simulink model "Winch_All_Controllers_with_Noise"  (R2016a)
settings: Solver=VariableStepAuto  SolverMode=SingleTasking  StartTime=0.0  StopTime=500  RelTol=1e-3
undefined symbols (not defined in the file or in its folder): K
libraries: mpclib x1, simulink x1
settings Model: Creator=shrenikzinage  LastModifiedBy=shrenikzinage
settings DataIOCC: SaveFormat=Array
settings DebuggingCC: SFUnexpectedBacktrackingDiag=error  SFNoUnconditionalDefaultTransitionDiag=error
settings SFSimCC: SimUseLocalCustomCode=on
settings RTWCC: RTWUseLocalCustomCode=on
settings GRTTargetCC: TargetLangStandard=C99 (ISO)  GeneratePreprocessorConditionals=Use local settings
settings ConfigComp: CovMetricSettings=dwe  CovHtmlReporting=off  CovSaveCumulativeToWorkspaceVar=off  CovSaveSingleToWorkspaceVar=off  CovExternalEMLEnable=on

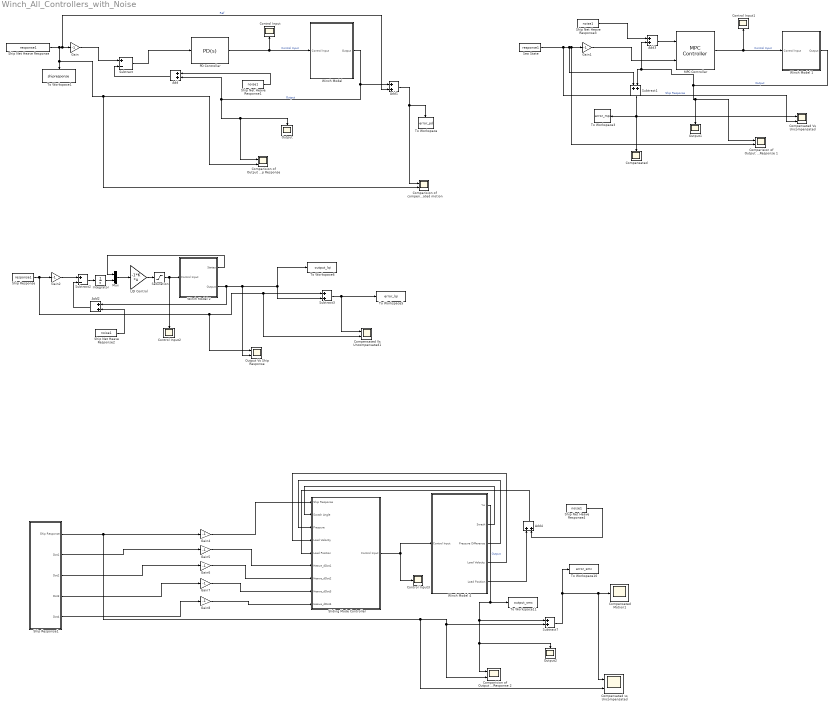
== system Winch_All_Controllers_with_Noise ==
  Add{,1..4} (5 alike) : Sum
  "Comparision of Output and Ship Response " : Scope  NumInputPorts=2
  Comparision of Output and Ship Response 1 : Scope  NumInputPorts=2
  Comparision of Output and Ship Response 2 : Scope  NumInputPorts=2
  Comparision of compensated and uncompensated motion : Scope  NumInputPorts=2
  Compensated : Scope
  Compensated Motion1 : Scope
  Compensated Vs Uncompensated : Scope  NumInputPorts=2
  Compensated Vs Uncompensated1 : Scope  NumInputPorts=2
  "Compensated vs Uncompensated " : Scope  NumInputPorts=2
  Control Input{,1..3} (4 alike) : Scope
  Gain{,1..2,4..8} (8 alike) : Gain  Gain=-1
  Integrator : Integrator
  LQI Control : Gain  Gain=-1*K  Multiplication=Matrix(K*u) (u vector)
  MPC Controller : mpclib/MPC Controller  SCDEnableBlockLinearizationSpecification=on  mpcobj=mpc1  is_multiple=0  enable_value=0  return_u0=off  updateMPCinCallerWorkspace=on  md_inport=off  mv_inport=off  uref_inport=off  cost_outport=off  return_sequence=off  return_qpstatus=off  return_xseq=off  return_state=off  return_ovseq=off  state_inport=off  umin_inport=off  umax_inport=off  ymin_inport=off  ymax_inport=off  cc_inport=off  ywt_inport=off  uwt_inport=off  duwt_inport=off  rhoeps_inport=off  pm_inport=off  MaximumP=10  HorizonChoice=FixedHorizon  n_ts=0.05  n_p=20  n_mv=1  n_md=0  n_ud=0  n_mo=1  n_uo=0  BlockDataType=double  SampleTimeInherited=off  switch_inport=off
  Mux : Mux  Inputs=2
  Output : Scope
  Output Vs Ship Response : Scope  NumInputPorts=2
  Output1 : Scope
  Output2 : Scope
  "PD Controller " : simulink/Continuous/PID Controller  Controller=PD  Form=Parallel  TimeDomain=Continuous-time  SampleTime=-1  IntegratorMethod=Forward Euler  FilterMethod=Forward Euler  ControllerParametersSource=internal  P=5.86  I=0.711  D=5.46  UseFilter=on  N=33.33  InitialConditionSource=internal  InitialConditionForIntegrator=0  InitialConditionForFilter=0  DifferentiatorICPrevScaledInput=0  ExternalReset=none  TrackingMode=off  Kt=1  LimitOutput=on  UpperSaturationLimit=200  LowerSaturationLimit=-200  LinearizeAsGain=on  AntiWindupMode=none  Kb=1  POutMin=[]  POutMax=[]  IOutMin=[]  IOutMax=[]  DOutMin=[]  DOutMax=[]  NOutMin=[]  NOutMax=[]  SumOutMin=[]  SumOutMax=[]  SaturationOutMin=[]  SaturationOutMax=[]  PParamMin=[]  PParamMax=[]  IParamMin=[]  IParamMax=[]  DParamMin=[]  DParamMax=[]  NParamMin=[]  NParamMax=[]  KbParamMin=[]  KbParamMax=[]  KtParamMin=[]  KtParamMax=[]  KbOutMin=[]  KbOutMax=[]  KtOutMin=[]  KtOutMax=[]  IntegratorOutMin=[]  IntegratorOutMax=[]  FilterOutMin=[]  FilterOutMax=[]  SumI1OutMin=[]  SumI1OutMax=[]  SumI2OutMin=[]  SumI2OutMax=[]  SumI3OutMin=[]  SumI3OutMax=[]  SumDOutMin=[]  SumDOutMax=[]  DifferentiatorOutMin=[]  DifferentiatorOutMax=[]  IntegratorContinuousStateAttributes=''  IntegratorStateMustResolveToSignalObject=off  IntegratorRTWStateStorageClass=Auto  FilterContinuousStateAttributes=''  FilterStateMustResolveToSignalObject=off  FilterRTWStateStorageClass=Auto
  Saturation : Saturate  UpperLimit=200  LowerLimit=-200
  Sea State : FromWorkspace  VariableName=response1  SampleTime=0
  Ship Net Heave Response : FromWorkspace  VariableName=response1  SampleTime=0
  Ship Net Heave Response{1..4} (4 alike) : FromWorkspace  VariableName=noise1  SampleTime=0
  Ship Response : FromWorkspace  VariableName=response1  SampleTime=0
  Ship Response1 : Subsystem
  Sliding Mode Controller : Subsystem
  Subtract : Sum  Inputs=+-
  Subtract1 : Sum
  Subtract2 : Sum  Inputs=+-
  Subtract3 : Sum
  Subtract7 : Sum
  To Workspace : ToWorkspace  VariableName=error_pd  SampleTime=-1
  To Workspace1 : ToWorkspace  VariableName=shipresponse  SampleTime=-1
  To Workspace10 : ToWorkspace  VariableName=error_smc  SampleTime=-1
  To Workspace11 : ToWorkspace  VariableName=output_smc  SampleTime=-1
  To Workspace3 : ToWorkspace  VariableName=error_mpc  SampleTime=-1
      settings: Save2DSignal=2-D array (concatenate along first dimension)
  To Workspace5 : ToWorkspace  VariableName=error_lqi  SampleTime=-1
  To Workspace6 : ToWorkspace  VariableName=output_lqi  SampleTime=-1
  "Winch Model " : Subsystem
  Winch Model 1 : Subsystem
  Winch Model 2 : Subsystem
  Winch Model 4 : Subsystem
  wires:
  LQI Control/1 -> Saturation/1
  Saturation/1 -> Winch Model 2/1(Control Input), Control Input2/1
  Ship Response1/4(Dot3) -> Gain7/1
  Winch Model 4/2(Swash) -> Sliding Mode Controller/2(Swash Angle)
  Winch Model 4/1(Yw) -> Comparision of Output and Ship Response 2/1, Output2/1, Subtract7/1, To Workspace11/1  "Output"
  Subtract7/1 -> To Workspace10/1, "Compensated vs Uncompensated "/1, Compensated Motion1/1
  Mux/1 -> LQI Control/1
  Gain8/1 -> Sliding Mode Controller/9(Heave_dDot4)
  Gain1/1 -> MPC Controller/2
  Ship Response1/3(Dot2) -> Gain6/1
  Winch Model 2/1(States) -> Mux/1
  Ship Response1/2(Dot1) -> Gain5/1
  Winch Model 4/3(Pressure Difference) -> Sliding Mode Controller/3(Pressure)
  Ship Response1/1(Ship Response) -> Gain4/1, "Compensated vs Uncompensated "/2, Comparision of Output and Ship Response 2/2, Subtract7/2
  Gain7/1 -> Sliding Mode Controller/8(Heave_dDot3)
  Ship Response1/5(Dot4) -> Gain8/1
  Subtract/1 -> "PD Controller "/1
  Gain5/1 -> Sliding Mode Controller/6("Heave_dDot1 ")
  Ship Response/1 -> Output Vs Ship Response/1, Compensated Vs Uncompensated1/2, Subtract3/1, Gain2/1
  Gain2/1 -> Subtract2/1
  Subtract2/1 -> Integrator/1
  Winch Model 1/1("Output ") -> Add3/2, Subtract1/2, Comparision of Output and Ship Response 1/1, Output1/1  "Output"
  Winch Model 4/4(Load Velocity) -> Sliding Mode Controller/4(Load Velocity)
  "PD Controller "/1 -> "Winch Model "/1(Control Input), Control Input/1  "Control Input"
  Integrator/1 -> Mux/2
  Winch Model 2/2("Output ") -> Add2/1, Output Vs Ship Response/2, Subtract3/2, To Workspace6/1
  Subtract3/1 -> Compensated Vs Uncompensated1/1, To Workspace5/1
  Gain/1 -> Subtract/1
  Sea State/1 -> Compensated Vs Uncompensated/2, Subtract1/1, Comparision of Output and Ship Response 1/2, Gain1/1  "Ship Response"
  Ship Net Heave Response/1 -> "Comparision of Output and Ship Response "/2, Comparision of compensated and uncompensated motion/2, To Workspace1/1, Add1/2, Gain/1  "Ref"
  MPC Controller/1 -> Winch Model 1/1("Control Input "), Control Input1/1  "Control Input"
  Sliding Mode Controller/1(Control Input) -> Winch Model 4/1(Control Input), Control Input3/1
  "Winch Model "/1("Output ") -> Add/2, "Comparision of Output and Ship Response "/1, Output/1, Add1/1  "Output"
  Subtract1/1 -> To Workspace3/1, Compensated/1, Compensated Vs Uncompensated/1
  Gain4/1 -> Sliding Mode Controller/1(Ship Response)
  Gain6/1 -> Sliding Mode Controller/7(Heave_dDot2)
  Ship Net Heave Response1/1 -> Add/1
  Add/1 -> Subtract/2
  Add1/1 -> To Workspace/1, Comparision of compensated and uncompensated motion/1
  Ship Net Heave Response2/1 -> Add2/2
  Add2/1 -> Subtract2/2
  Ship Net Heave Response3/1 -> Add3/1
  Add3/1 -> MPC Controller/1
  Winch Model 4/5(Load Position) -> Add4/1
  Ship Net Heave Response4/1 -> Add4/2
  Add4/1 -> Sliding Mode Controller/5(Load Position)

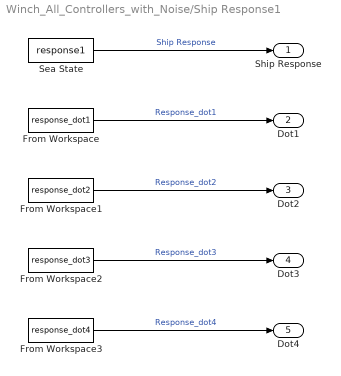
== system Winch_All_Controllers_with_Noise/Ship Response1 ==
  From Workspace : FromWorkspace  VariableName=response_dot1  SampleTime=0
  From Workspace1 : FromWorkspace  VariableName=response_dot2  SampleTime=0
  From Workspace2 : FromWorkspace  VariableName=response_dot3  SampleTime=0
  From Workspace3 : FromWorkspace  VariableName=response_dot4  SampleTime=0
  "Sea State " : FromWorkspace  VariableName=response1  SampleTime=0
  Ship Response : Outport
  Dot1 : Outport  Port=2
  Dot2 : Outport  Port=3
  Dot3 : Outport  Port=4
  Dot4 : Outport  Port=5
  wires:
  "Sea State "/1 -> Ship Response/1  "Ship Response"
  From Workspace3/1 -> Dot4/1  "Response_dot4"
  From Workspace1/1 -> Dot2/1  "Response_dot2"
  From Workspace2/1 -> Dot3/1  "Response_dot3"
  From Workspace/1 -> Dot1/1  "Response_dot1"

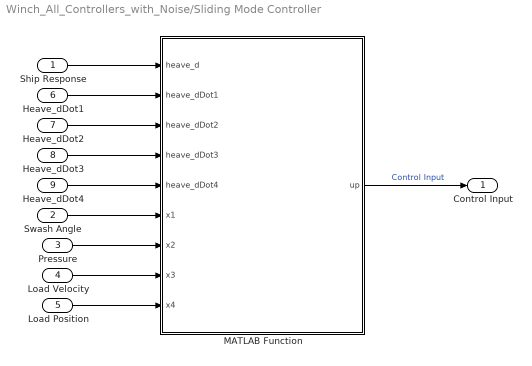
== system Winch_All_Controllers_with_Noise/Sliding Mode Controller ==
  Ship Response : Inport
  Swash Angle : Inport  Port=2
  Pressure : Inport  Port=3
  Load Velocity : Inport  Port=4
  Load Position : Inport  Port=5
  "Heave_dDot1 " : Inport  Port=6
  Heave_dDot2 : Inport  Port=7
  Heave_dDot3 : Inport  Port=8
  Heave_dDot4 : Inport  Port=9
  MATLAB Function : MATLAB Function  TreatAsAtomicUnit=on
  Control Input : Outport
  wires:
  Heave_dDot4/1 -> MATLAB Function/5(heave_dDot4)
  Ship Response/1 -> MATLAB Function/1(heave_d)
  MATLAB Function/1(up) -> Control Input/1  "Control Input"
  Heave_dDot2/1 -> MATLAB Function/3(heave_dDot2)
  Load Velocity/1 -> MATLAB Function/8(x3)
  Heave_dDot3/1 -> MATLAB Function/4(heave_dDot3)
  Load Position/1 -> MATLAB Function/9(x4)
  "Heave_dDot1 "/1 -> MATLAB Function/2(heave_dDot1)
  Swash Angle/1 -> MATLAB Function/6(x1)
  Pressure/1 -> MATLAB Function/7(x2)

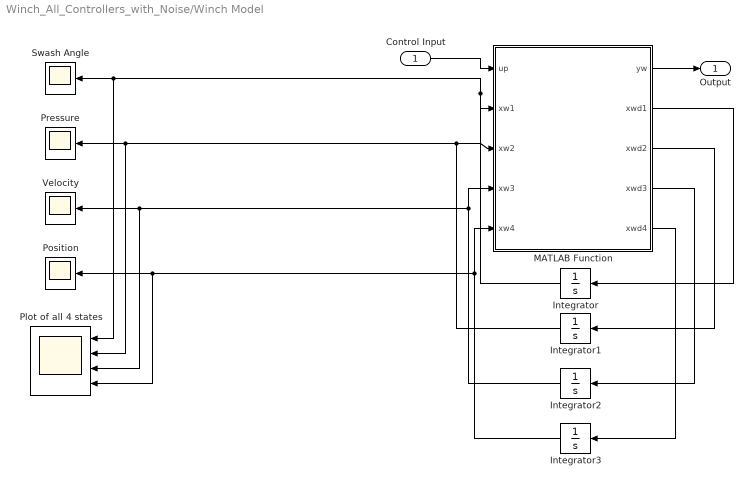
== system Winch_All_Controllers_with_Noise/Winch Model  ==
  Control Input : Inport
  Integrator : Integrator  InitialCondition=0.4  LimitOutput=on  UpperSaturationLimit=1  LowerSaturationLimit=-1  ContinuousStateAttributes='Swash'
  Integrator1 : Integrator  InitialCondition=188e5  UpperSaturationLimit=4e7  LowerSaturationLimit=-4e7  ContinuousStateAttributes='Pressure'
  Integrator2 : Integrator  ContinuousStateAttributes='Velocity'
  Integrator3 : Integrator  ContinuousStateAttributes='Position'
  MATLAB Function : MATLAB Function  TreatAsAtomicUnit=on
  Plot of all 4 states : Scope  NumInputPorts=4
  Position : Scope
  Pressure : Scope
  Swash Angle : Scope
  Velocity : Scope
  "Output " : Outport
  wires:
  Integrator2/1 -> MATLAB Function/4(xw3), Plot of all 4 states/3, Velocity/1
  MATLAB Function/4(xwd3) -> Integrator2/1
  MATLAB Function/3(xwd2) -> Integrator1/1
  Integrator/1 -> Plot of all 4 states/1, Swash Angle/1, MATLAB Function/2(xw1)
  MATLAB Function/2(xwd1) -> Integrator/1
  Integrator1/1 -> MATLAB Function/3(xw2), Plot of all 4 states/2, Pressure/1
  Integrator3/1 -> MATLAB Function/5(xw4), Plot of all 4 states/4, Position/1
  Control Input/1 -> MATLAB Function/1(up)
  MATLAB Function/5(xwd4) -> Integrator3/1
  MATLAB Function/1(yw) -> "Output "/1

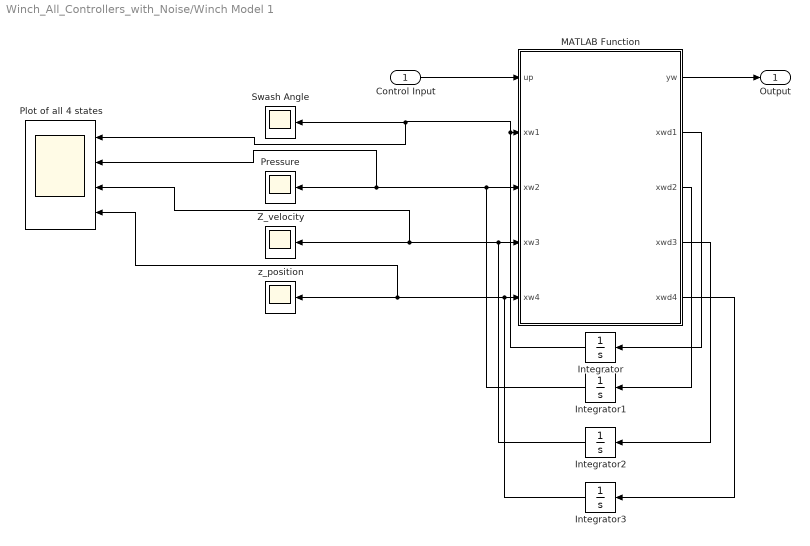
== system Winch_All_Controllers_with_Noise/Winch Model 1 ==
  "Control Input " : Inport
  Integrator : Integrator  InitialCondition=0.3  LimitOutput=on  UpperSaturationLimit=1  LowerSaturationLimit=-1
  Integrator1 : Integrator  InitialCondition=188e5  UpperSaturationLimit=5e7  LowerSaturationLimit=-5e7
  Integrator2 : Integrator
  Integrator3 : Integrator
  MATLAB Function : MATLAB Function  TreatAsAtomicUnit=on
  Plot of all 4 states : Scope  NumInputPorts=4
  Pressure : Scope
  Swash Angle : Scope
  Z_velocity : Scope
  z_position : Scope
  "Output " : Outport
  wires:
  MATLAB Function/1(yw) -> "Output "/1
  Integrator2/1 -> MATLAB Function/4(xw3), Z_velocity/1, Plot of all 4 states/3
  MATLAB Function/4(xwd3) -> Integrator2/1
  MATLAB Function/3(xwd2) -> Integrator1/1
  Integrator/1 -> Plot of all 4 states/1, Swash Angle/1, MATLAB Function/2(xw1)
  MATLAB Function/2(xwd1) -> Integrator/1
  Integrator1/1 -> MATLAB Function/3(xw2), Plot of all 4 states/2, Pressure/1
  Integrator3/1 -> MATLAB Function/5(xw4), Plot of all 4 states/4, z_position/1
  "Control Input "/1 -> MATLAB Function/1(up)
  MATLAB Function/5(xwd4) -> Integrator3/1

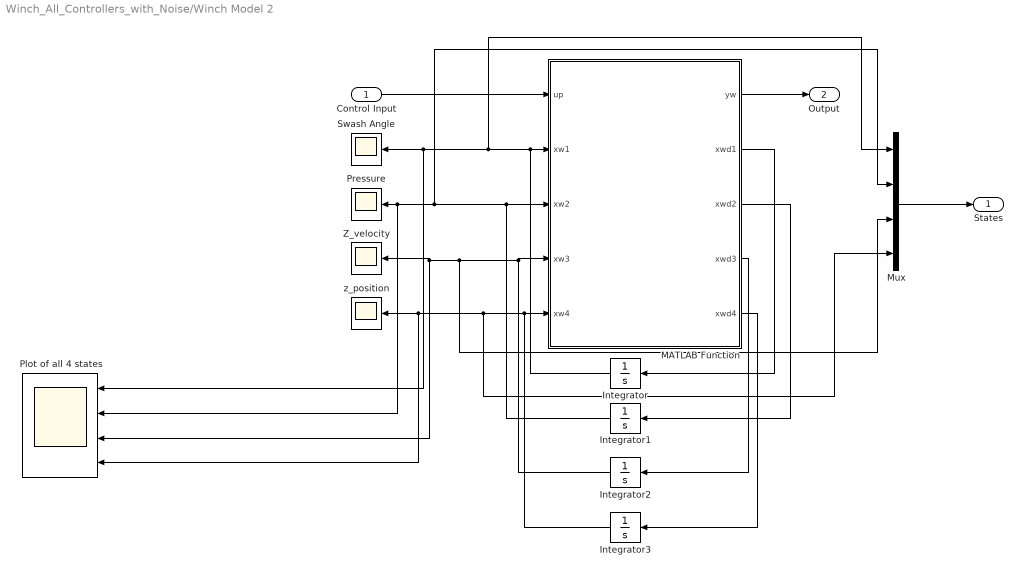
== system Winch_All_Controllers_with_Noise/Winch Model 2 ==
  Control Input : Inport
  Integrator : Integrator  InitialCondition=0.3  LimitOutput=on  UpperSaturationLimit=1  LowerSaturationLimit=-1
  Integrator1 : Integrator  InitialCondition=188e5  UpperSaturationLimit=5e7  LowerSaturationLimit=-5e7
  Integrator2 : Integrator
  Integrator3 : Integrator
  MATLAB Function : MATLAB Function  TreatAsAtomicUnit=on
  Mux : Mux
  Plot of all 4 states : Scope  NumInputPorts=4
  Pressure : Scope
  Swash Angle : Scope
  Z_velocity : Scope
  z_position : Scope
  States : Outport
  "Output " : Outport  Port=2
  wires:
  Integrator2/1 -> MATLAB Function/4(xw3), Mux/3, Z_velocity/1, Plot of all 4 states/3
  MATLAB Function/4(xwd3) -> Integrator2/1
  MATLAB Function/3(xwd2) -> Integrator1/1
  Integrator/1 -> Mux/1, Swash Angle/1, Plot of all 4 states/1, MATLAB Function/2(xw1)
  MATLAB Function/2(xwd1) -> Integrator/1
  Integrator1/1 -> MATLAB Function/3(xw2), Mux/2, Plot of all 4 states/2, Pressure/1
  Integrator3/1 -> MATLAB Function/5(xw4), z_position/1, Plot of all 4 states/4, Mux/4
  Control Input/1 -> MATLAB Function/1(up)
  MATLAB Function/5(xwd4) -> Integrator3/1
  Mux/1 -> States/1
  MATLAB Function/1(yw) -> "Output "/1

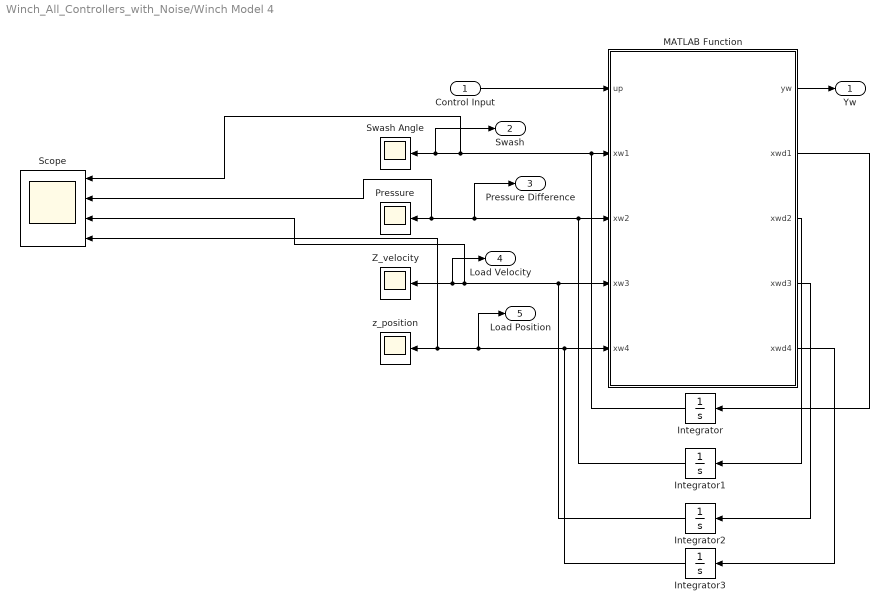
== system Winch_All_Controllers_with_Noise/Winch Model 4 ==
  Control Input : Inport
  Integrator : Integrator  InitialCondition=0.3  LimitOutput=on  UpperSaturationLimit=1  LowerSaturationLimit=-1
  Integrator1 : Integrator  InitialCondition=188e5  UpperSaturationLimit=5e7  LowerSaturationLimit=-5e7
  Integrator2 : Integrator
  Integrator3 : Integrator
  MATLAB Function : MATLAB Function  TreatAsAtomicUnit=on
  Pressure : Scope
  Scope : Scope  NumInputPorts=4
  Swash Angle : Scope
  Z_velocity : Scope
  z_position : Scope
  Yw : Outport
  Swash : Outport  Port=2
  Pressure Difference : Outport  Port=3
  Load Velocity : Outport  Port=4
  Load Position : Outport  Port=5
  wires:
  MATLAB Function/1(yw) -> Yw/1
  MATLAB Function/4(xwd3) -> Integrator2/1
  MATLAB Function/3(xwd2) -> Integrator1/1
  MATLAB Function/2(xwd1) -> Integrator/1
  Control Input/1 -> MATLAB Function/1(up)
  MATLAB Function/5(xwd4) -> Integrator3/1
  Integrator/1 -> Scope/1, Swash/1, Swash Angle/1, MATLAB Function/2(xw1)
  Integrator2/1 -> Load Velocity/1, Z_velocity/1, Scope/3, MATLAB Function/4(xw3)
  Integrator3/1 -> Load Position/1, Scope/4, z_position/1, MATLAB Function/5(xw4)
  Integrator1/1 -> Pressure Difference/1, Scope/2, Pressure/1, MATLAB Function/3(xw2)

== matlab function Winch_All_Controllers_with_Noise/Winch Model 1/MATLAB Function ==
  data: up input; yw output; xw1 input; xw2 input; xw3 input; xw4 input; xwd1 output; xwd2 output; xwd3 output; xwd4 output
function  [yw,xwd1,xwd2,xwd3,xwd4]= winch(up,xw1,xw2,xw3,xw4)


g = 9.81;                   % Acceleration due to gravity
k_oil = 1.8e9;              % Bulk Modulus of Mineral Oil in Pa
Vc = 2e-3;                  % Volume of the hydraulic lines in m^3
Dp = 40e-6;                  % Maximum Pump Displacment in m^3
Dm = 4e-6;                   % Fixed Displacement Motor in m^3
w_p = 45;                   % Rotation rate of Pump in Hz
Tp = 1;                    % Time constant
k = 200;                    % Gear transmission ratio
r = 0.5;                    % Radius of Winch
eta_m = 0.65;               % Efficency of motor
Jw = 150;                   % Inertia of the winch
d = 1e4;                    % Viscous friction of winch
m = 1e3;                   % Mass load(Fixed)

% up_bar = -(k1p + k1m)*m*g*r/(k*Dm*Dp*w_p);
% zwd_max = r*k*Dm*Dp*eta_m*w_p / ((k1p + k1m)*d + (Dm*k)^2*eta_m);

% Matrices %

A = [-1/Tp 0 0 0;
      (-2*k_oil/Vc)*Dp*w_p 0 (2*k_oil/Vc)*Dm*k/r 0;
      0 -r/(Jw + m*r^2)*Dm*k*eta_m -d/(Jw + m*r^2) 0;
      0 0 1 0;];

B = [1/Tp 0 0 0]';

ew = [0 0 (r^2)*m*g/(Jw + m*(r^2)) 0]';

C = [0 0 0 1];

xw = [xw1;xw2;xw3;xw4];

% up = uw/zwd_max + up_bar ;

% State Space Equation

xwd = A*xw + B*up ;

% States

xwd1 = xwd(1);
xwd2 = xwd(2);
xwd3 = xwd(3);
xwd4 = xwd(4);

% Output

yw = xw(4);

end

== matlab function Winch_All_Controllers_with_Noise/Winch Model /MATLAB Function ==
  data: up input; yw output; xw1 input; xw2 input; xw3 input; xw4 input; xwd1 output; xwd2 output; xwd3 output; xwd4 output
function  [yw,xwd1,xwd2,xwd3,xwd4]= pd(up,xw1,xw2,xw3,xw4)

g = 9.81;                   % Acceleration due to gravity
k_oil = 1.8e9;              % Bulk Modulus of Mineral Oil in Pa
Vc = 2e-3;                  % Volume of the hydraulic lines in m^3
Dp = 40e-6;                  % Maximum Pump Displacment in m^3
Dm = 4e-6;                   % Fixed Displacement Motor in m^3
w_p = 45;                   % Rotation rate of Pump in Hz
Tp = 1;                    % Time constant
k = 200;                    % Gear transmission ratio
r = 0.5;                    % Radius of Winch
eta_m = 0.65;               % Efficency of motor
Jw = 150;                   % Inertia of the winch
d = 1e4;                    % Viscous friction of winch
m = 1e3;                   % Mass load(Fixed)

%---

% up_bar = -(k1p + k1m)*m*g*r/(k*Dm*Dp*w_p);
% zwd_max = r*k*Dm*Dp*eta_m*w_p / ((k1p + k1m)*d + (Dm*k)^2*eta_m);

% ----- 

% State Space Matrices %

A = [-1/Tp 0 0 0;
      (-2*k_oil/Vc)*(Dp*w_p) 0 (2*k_oil/Vc)*(Dm*k/r) 0;
      0 -(r/(Jw + m*r^2))*(Dm*k*eta_m) -d/(Jw + m*r^2) 0;
      0 0 1 0;];

B = [1/Tp 0 0 0]';

e = [0 0 (r^2)*m*g/(Jw + m*(r^2)) 0]';

C = [0 0 0 1];

xw = [xw1;xw2;xw3;xw4];

% up = uw/zwd_max + up_bar ;

% Linear State Space Equation

xwd = A*xw + B*up;

% States

xwd1 = xwd(1);
xwd2 = xwd(2);
xwd3 = xwd(3);
xwd4 = xwd(4);

% Output

yw = xw(4);

end

== matlab function Winch_All_Controllers_with_Noise/Winch Model 2/MATLAB Function ==
  data: yw output; up input; xw1 input; xw2 input; xw3 input; xw4 input; xwd1 output; xwd2 output; xwd3 output; xwd4 output
function  [yw,xwd1,xwd2,xwd3,xwd4]= lqi(up,xw1,xw2,xw3,xw4)

g = 9.81;                   % Acceleration due to gravity
k_oil = 1.8e9;              % Bulk Modulus of Mineral Oil in Pa
Vc = 2e-3;                  % Volume of the hydraulic lines in m^3
Dp = 40e-6;                  % Maximum Pump Displacment in m^3
Dm = 4e-6;                   % Fixed Displacement Motor in m^3
w_p = 45;                   % Rotation rate of Pump in Hz
Tp = 1;                    % Time constant
k = 200;                    % Gear transmission ratio
r = 0.5;                    % Radius of Winch
eta_m = 0.65;               % Efficency of motor
Jw = 150;                   % Inertia of the winch
d = 1e4;                    % Viscous friction of winch
m = 1e3;                   % Mass load(Fixed)

% up_bar = -(k1p + k1m)*m*g*r/(k*Dm*Dp*w_p);
% zwd_max = r*k*Dm*Dp*eta_m*w_p / ((k1p + k1m)*d + (Dm*k)^2*eta_m);


% Matrices %

A = [-1/Tp 0 0 0;
      (-2*k_oil/Vc)*Dp*w_p 0 (2*k_oil/Vc)*Dm*k/r 0;
      0 -r/(Jw + m*r^2)*Dm*k*eta_m -d/(Jw + m*r^2) 0;
      0 0 1 0;];

B = [1/Tp 0 0 0]';

ew = [0 0 (r^2)*m*g/(Jw + m*(r^2)) 0]';

C = [0 0 0 1];

xw = [xw1;xw2;xw3;xw4];

% up = uw/zwd_max + up_bar ;

% State Space Equation

xwd = A*xw + B*up ;

% States
xwd1 = xwd(1);
xwd2 = xwd(2);
xwd3 = xwd(3);
xwd4 = xwd(4);

% Output
yw = xw4;

end

== matlab function Winch_All_Controllers_with_Noise/Sliding Mode Controller/MATLAB Function ==
  data: heave_d input; up output; heave_dDot1 input; heave_dDot2 input; heave_dDot3 input; heave_dDot4 input; x1 input; x2 input; x3 input; x4 input
function up  = sliding(heave_d,heave_dDot1,heave_dDot2,heave_dDot3,heave_dDot4,x1,x2,x3,x4)


g = 9.81;                   % Acceleration due to gravity
k_oil = 1.8e9;              % Bulk Modulus of Mineral Oil in Pa
Vc = 2e-3;                  % Volume of the hydraulic lines in m^3
Dp = 40e-6;                  % Maximum Pump Displacment in m^3
Dm = 4e-6;                   % Fixed Displacement Motor in m^3
w_p = 45;                   % Rotation rate of Pump in Hz
k1p = 0;                % Leakage Constant for pump(Fixed)
k1m = 0;                % Leakage Constant for Motor(Fixed)
Tp = 1;                    % Time constant
k = 200;                    % Gear transmission ratio
r = 0.5;                    % Radius of Winch
eta_m = 0.65;               % Efficency of motor
Jw = 150;                   % Inertia of the winch
d = 1e4;                    % Viscous friction of winch
m = 1e3;                   % Mass load(Fixed)

% up_bar = -(k1p + k1m)*m*g*r/(k*Dm*Dp*w_p);
% zwd_max = r*k*Dm*Dp*eta_m*w_p / ((k1p + k1m)*d + (Dm*k)^2*eta_m);

%---

A = [-1/Tp 0 0 0;
      (-2*k_oil/Vc)*Dp*w_p 0 (2*k_oil/Vc)*Dm*k/r 0;
      0 -r/(Jw + m*r^2)*Dm*k*eta_m -d/(Jw + m*r^2) 0;
      0 0 1 0;];

B = [1/Tp 0 0 0]';

ew = [0 0 r^2*m*g/(Jw + m*r^2) 0]';

C = [0 0 0 1];

% Control Parameters

kp = 70;
lambda = 27; 

k3 = (lambda)^3;
k2 = 3*(lambda)^2;
k1 = 3*lambda;


%---- Control Input

S = heave_dDot3 + k2*(heave_dDot1 - x3) + k3*(heave_d - x4) + k1*(heave_dDot2 + (d*x3)/(m*r^2 + Jw) + (Dm*eta_m*k*r*x2)/(m*r^2 + Jw)) - (d*((d*x3)/(m*r^2 + Jw) + (Dm*eta_m*k*r*x2)/(m*r^2 + Jw)))/(m*r^2 + Jw) - (Dm*eta_m*k*r*((2*k_oil*x2*(k1m + k1p))/Vc + (2*Dp*k_oil*w_p*x1)/Vc - (2*Dm*k*k_oil*x3)/(Vc*r)))/(m*r^2 + Jw);

up = heave_dDot4 + kp*sign(S) + ((Dm*d*eta_m*k*r)/(m*r^2 + Jw)^2 + (2*Dm*eta_m*k*k_oil*r*(k1m + k1p))/(Vc*(m*r^2 + Jw)))*((2*k_oil*x2*(k1m + k1p))/Vc + (2*Dp*k_oil*w_p*x1)/Vc - (2*Dm*k*k_oil*x3)/(Vc*r)) + k3*(heave_dDot1 - x3) + k2*(heave_dDot2 + (d*x3)/(m*r^2 + Jw) + (Dm*eta_m*k*r*x2)/(m*r^2 + Jw)) + (d^2/(m*r^2 + Jw)^2 - (2*Dm^2*eta_m*k^2*k_oil)/(Vc*(m*r^2 + Jw)))*((d*x3)/(m*r^2 + Jw) + (Dm*eta_m*k*r*x2)/(m*r^2 + Jw)) - k1*((d*((d*x3)/(m*r^2 + Jw) + (Dm*eta_m*k*r*x2)/(m*r^2 + Jw)))/(m*r^2 + Jw) - heave_dDot3 + (Dm*eta_m*k*r*((2*k_oil*x2*(k1m + k1p))/Vc + (2*Dp*k_oil*w_p*x1)/Vc - (2*Dm*k*k_oil*x3)/(Vc*r)))/(m*r^2 + Jw)) + (2*Dm*Dp*eta_m*k*k_oil*r*w_p*x1)/(Tp*Vc*(m*r^2 + Jw));
 
end

== matlab function Winch_All_Controllers_with_Noise/Winch Model 4/MATLAB Function ==
  data: up input; yw output; xw1 input; xw2 input; xw3 input; xw4 input; xwd1 output; xwd2 output; xwd3 output; xwd4 output
function  [yw,xwd1,xwd2,xwd3,xwd4]= winch(up,xw1,xw2,xw3,xw4)

g = 9.81;                   % Acceleration due to gravity
k_oil = 1.8e9;              % Bulk Modulus of Mineral Oil in Pa
Vc = 2e-3;                  % Volume of the hydraulic lines in m^3
Dp = 40e-6;                  % Maximum Pump Displacment in m^3
Dm = 4e-6;                   % Fixed Displacement Motor in m^3
w_p = 45;                   % Rotation rate of Pump in Hz
Tp = 1;                    % Time constant
k = 200;                    % Gear transmission ratio
r = 0.5;                    % Radius of Winch
eta_m = 0.65;               % Efficency of motor
Jw = 150;                   % Inertia of the winch
d = 1e4;                    % Viscous friction of winch
m = 1e3;                   % Mass load(Fixed)

% up_bar = -(k1p + k1m)*m*g*r/(k*Dm*Dp*w_p);
% zwd_max = r*k*Dm*Dp*eta_m*w_p / ((k1p + k1m)*d + (Dm*k)^2*eta_m);


% Matrices %

A = [-1/Tp 0 0 0;
      (-2*k_oil/Vc)*Dp*w_p 0 (2*k_oil/Vc)*Dm*k/r 0;
      0 -r/(Jw + m*r^2)*Dm*k*eta_m -d/(Jw + m*r^2) 0;
      0 0 1 0;];

B = [1/Tp 0 0 0]';

ew = [0 0 (r^2)*m*g/(Jw + m*(r^2)) 0]';

C = [0 0 0 1];

xw = [xw1;xw2;xw3;xw4];

% State Space Equation
xwd = A*xw + B*up;

% States
xwd1 = xwd(1);
xwd2 = xwd(2);
xwd3 = xwd(3);
xwd4 = xwd(4);

% Output
yw = xw(4);

end
